simulink model "PMSM_PI_T"  (R2016a)
settings: Solver=ode23tb  StartTime=0.0  StopTime=1.4  FixedStep=Ts  MaxStep=0.0001  RelTol=1e-4
InitFcn:
  | Ts = 10e-6;
  | 
  | R = 0.958;
  | Ld = 5.25e-3;
  | Lq = 12e-3;
  | Pn = 4;
  | flux = 0.1827;
undefined symbols (not defined in the file): DiscIntNeverNeededParam
libraries: powerlib x13, simulink x2, powerlib_extras x2
settings Model: Creator=SUN  LastModifiedBy=Administrator
settings SolverCC: ZeroCrossControl=DisableAll
settings DataIOCC: LimitDataPoints=on  SaveFormat=Array  SignalLoggingSaveFormat=ModelDataLogs
settings OptimizationCC: ExpressionDepthLimit=2147483647  InitFltsAndDblsToZero=on
settings DebuggingCC: UnderspecifiedInitializationDetection=Classic  MergeDetectMultiDrivingBlocksExec=none  SolverPrmCheckMsg=warning  FcnCallInpInsideContextMsg=UseLocalSettings  StateNameClashWarn=warning
settings HardwareCC: ProdBitPerPointer=32  ProdLargestAtomicFloat=None  ProdIntDivRoundTo=Undefined  ProdEndianess=Unspecified  ProdWordSize=32  ProdHWDeviceType=32-bit Generic
settings ModelReferenceCC: PropagateSignalLabelsOutOfModel=off
settings GRTTargetCC: CombineOutputUpdateFcns=off  GRTInterface=on
settings ConfigComp: CovModelRefEnable=Off  CovSFcnEnable=off

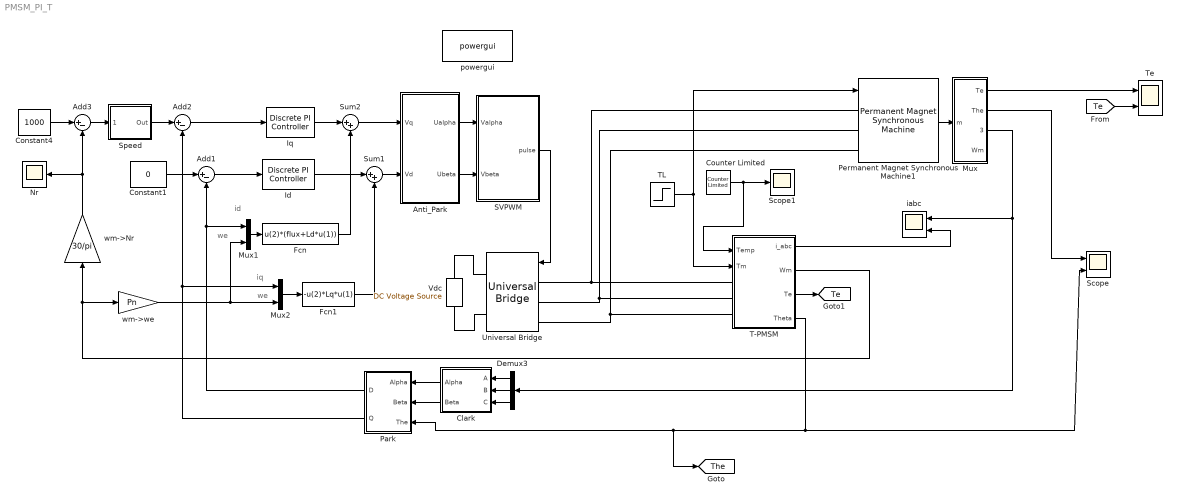
== system PMSM_PI_T ==
  note: iq
  note: we
  note: we
  note: id
  Add1 : Sum  Inputs=|+-
  Add2 : Sum  Inputs=|+-
  Add3 : Sum  Inputs=|+-
  Anti_Park : Subsystem
  Clark : Subsystem
  Constant1 : Constant  Value=0
  Constant4 : Constant  Value=1000
  Counter Limited : simulink/Sources/Counter Limited  uplimit=150  tsamp=0.0093
  Demux3 : Demux  Outputs=3
  Fcn : Fcn  Expr=u(2)*(flux+Ld*u(1))
  Fcn1 : Fcn  Expr=-u(2)*Lq*u(1)
  Id : powerlib_extras/Discrete  Control Blocks/Discrete PI Controller  Kp=Ld*1100  Ki=R*1100  Par_Limits=[311*0.9*sqrt(1/3) -311*0.9*sqrt(1/3)]  Init=0  Ts=Ts
  Iq : powerlib_extras/Discrete  Control Blocks/Discrete PI Controller  Kp=Lq*1100  Ki=R*1100  Par_Limits=[311*0.9*sqrt(1/3) -311*0.9*sqrt(1/3)]  Init=0  Ts=Ts
  Mux : Subsystem
  Mux1 : Mux  Inputs=2
  Mux2 : Mux  Inputs=2
  Nr : Scope
  Park : Subsystem
  Permanent Magnet Synchronous Machine1 : powerlib/Machines/Permanent Magnet Synchronous Machine  NbPhases=3  FluxDistribution=Sinusoidal  RotorType=Salient-pole  MechanicalLoad=Torque Tm  PresetModel=No  ShowDetailedParameters=on  MeasurementBus=off  Resistance=0.958  Inductance=8.5e-3  dqInductances=[5.25e-3,12e-3]  La=0.000835  MachineConstant=Flux linkage established by magnets (V.s)  Flux=0.1827  VoltageCst=132.5525  TorqueCst=1.0962  Flat=120  Mechanical=[0.003 0.008 4]  PolePairs=3  InitialConditions=[0,0, 0,0]  InitialConditions5ph=[0 0 0 0 0 0]  TsPowergui=0  TsBlock=-1  RefAngle=Aligned with phase A axis (original Park)
  SVPWM : Subsystem
  Scope : Scope  NumInputPorts=2
  Scope1 : Scope
  Speed : Subsystem  AncestorBlock=|  DialogController=POWERSYS.PowerSysDialog  mask(Discrete PI Controller){Kpw=0.14, Kiw=0.14*50, Ba=0.013, Par_Limits=[30 -30], Init=0, Ts=Ts}
      | powerlib_extras/Discrete 
      | Control Blocks/Discrete
      | PI Controller
      mask prompts: Kpw "Proportional gain (Kp):"; Kiw "Integral gain (Ki):"; Ba "feedback gain (Ba)"; Par_Limits "Output limits: [ Upper   Lower ]"; Init "Output initial value:"; Ts "Sample time:"
      mask help: This block implements a discrete PI controller.
      mask init:
      | UpperLimit=Par_Limits(1);
      | LowerLimit=Par_Limits(2);
      | power_initmask();
      mask Help: This block is part of a subset of blocks in the Extras library that does not have documentation associated with it, other than the block mask description.
      mask Display: disp('PI');
  Sum1 : Sum  Inputs=|++
  Sum2 : Sum  Inputs=|++
  T-PMSM : Subsystem
  TL : Step  Time=0.2  After=10  SampleTime=0
  Te : Scope  NumInputPorts=2
  Universal Bridge : powerlib/Power Electronics/Universal Bridge  Arms=3  SnubberResistance=1e5  SnubberCapacitance=inf  Device=IGBT / Diodes  Ron=1e-3  Lon=0  ForwardVoltages="[  0  0  ]"  ForwardVoltage=0  GTOparameters=[ 10e-6 , 20e-6 ]  IGBTparameters=[ 1e-6 , 2e-6 ]  Measurements=None  Measurements_2=None  converterType=Rectifier
  Vdc : powerlib/Electrical Sources/DC Voltage Source  Amplitude=311  Measurements=None
  iabc : Scope  NumInputPorts=2
  powergui : powerlib/powergui  SimulationMode=Continuous  SolverType=Tustin/Backward Euler (TBE)  SampleTime=Ts  frequency=60  SPID=off  DisableSnubberDevices=off  DisableRonSwitches=off  DisableVfSwitches=off  SwTol=0  DisplayEquations=off  Interpol=off  ExternalGateDelay=off  methode=off  Ts=0  FunctionMessages=off  echomessages=off  HookPort=off  EnableUseOfTLC=off  x0status=blocks  frequencyindice=0  Pbase=100e6  ErrMax=1e-4  Iterations=50  UnitsV=kV  UnitsW=MW  buscounter=0  RestoreLinks=warning  ResistiveCurrentMeasurement=off  Frange=[0:2:500]  Ylog=off  Xlog=on  ShowGrid=off  save=off  variable=ZData  structure=0  ZoomFFT=on  StartTime=0.0  cycles=1  DisplayStyle=1  fundamental=60  FreqAxis=off  MaxFrequency=1000  frequencyindicesteady=1  RmsSteady=1  display=off
  wm->Nr : Gain  Gain=30/pi
  wm->we : Gain  Gain=Pn
  tag scope: Te=global, The=global
  wires:
  TL/1 -> Permanent Magnet Synchronous Machine1/1, T-PMSM/2(Tm)
  Permanent Magnet Synchronous Machine1/1 -> Mux/1(m)
  Add3/1 -> Speed/1(Error)
  Constant4/1 -> Add3/1
  Fcn/1 -> Sum2/2
  Fcn1/1 -> Sum1/2
  Constant1/1 -> Add1/1
  Add1/1 -> Id/1
  wm->Nr/1 -> Add3/2, Nr/1
  Id/1 -> Sum1/1
  wm->we/1 -> Mux2/2, Mux1/2
  Mux1/1 -> Fcn/1
  Mux2/1 -> Fcn1/1
  Speed/1(Out) -> Add2/1
  Add2/1 -> Iq/1
  Iq/1 -> Sum2/1
  Sum2/1 -> Anti_Park/1(Vq)
  Sum1/1 -> Anti_Park/2(Vd)
  Mux/2(The) -> Scope/1
  SVPWM/1(pulse) -> Universal Bridge/1
  Mux/3(Iabc) -> Demux3/1, iabc/1
  Anti_Park/1(Ualpha) -> SVPWM/1(Valpha)
  Anti_Park/2(Ubeta) -> SVPWM/2(Vbeta)
  Clark/1(Alpha) -> Park/1(Alpha)
  Demux3/1 -> Clark/1(A)
  Demux3/2 -> Clark/2(B)
  Demux3/3 -> Clark/3(C)
  Clark/2(Beta) -> Park/2(Beta)
  Park/1(D) -> Mux1/1, Add1/2
  Park/2(Q) -> Mux2/1, Add2/2
  T-PMSM/1(i_abc) -> iabc/2
  T-PMSM/2(Wm) -> wm->we/1, wm->Nr/1
  T-PMSM/4(Theta) -> [The], Park/3(The), Scope/2
  T-PMSM/3(Te) -> [Te]
  [Te] -> Te/2
  Counter Limited/1 -> T-PMSM/1(Temp), Scope1/1
  Mux/1(Te) -> Te/1
  connections:
  Universal Bridge/RConn1 -- Vdc/RConn1
  Universal Bridge/RConn2 -- Vdc/LConn1
  Permanent Magnet Synchronous Machine1/LConn1 -- T-PMSM/LConn1 -- Universal Bridge/LConn1
  Permanent Magnet Synchronous Machine1/LConn2 -- Universal Bridge/LConn2 -- T-PMSM/LConn2
  Permanent Magnet Synchronous Machine1/LConn3 -- Universal Bridge/LConn3 -- T-PMSM/LConn3

== system PMSM_PI_T/Anti_Park ==
  Vq : Inport
  Vd : Inport  Port=2
  Fcn : Fcn  Expr=cos(u[1])*u[2]-sin(u[1])*u[3]
  Fcn1 : Fcn  Expr=sin(u[1])*u[2]+cos(u[1])*u[3]
  Mux1 : Mux  Inputs=3
  Ualpha : Outport
  Ubeta : Outport  Port=2
  wires:
  Fcn1/1 -> Ubeta/1
  Fcn/1 -> Ualpha/1
  Mux1/1 -> Fcn/1, Fcn1/1
  Vd/1 -> Mux1/2
  Vq/1 -> Mux1/3
  [The] -> Mux1/1

== system PMSM_PI_T/Clark ==
  A : Inport
  B : Inport  Port=2
  C : Inport  Port=3
  Mux : Mux  Inputs=3
  alpha : Fcn  Expr=(u(1)-0.5*(u(2)+u(3)))*2/3
  beta : Fcn  Expr=sqrt(3)/2*(u(2)-u(3))*2/3
  Alpha : Outport
  Beta : Outport  Port=2
  wires:
  alpha/1 -> Alpha/1
  B/1 -> Mux/2
  C/1 -> Mux/3
  A/1 -> Mux/1
  Mux/1 -> beta/1, alpha/1
  beta/1 -> Beta/1

== system PMSM_PI_T/Mux ==
  m : Inport
  Bus Selector : BusSelector  OutputSignals=Stator current is_a (A),Stator current is_b (A),Stator current is_c (A)
  Bus Selector1 : BusSelector  OutputSignals=Rotor speed wm (rad/s),Rotor angle thetam (rad),Electromagnetic torque Te (N*m)
  Mux : Mux  Inputs=3
  Te : Outport
  The : Outport  Port=2
  Iabc : Outport  Port=3
  Wm : Outport  Port=4
  wires:
  Bus Selector1/1 -> Wm/1  "<Rotor speed wm (rad/s)>"
  Bus Selector1/2 -> The/1  "<Rotor angle thetam (rad)>"
  Bus Selector1/3 -> Te/1  "<Electromagnetic torque Te (N*m)>"
  m/1 -> Bus Selector/1, Bus Selector1/1
  Bus Selector/2 -> Mux/2  "<Stator current is_b (A)>"
  Bus Selector/3 -> Mux/3  "<Stator current is_c (A)>"
  Bus Selector/1 -> Mux/1  "<Stator current is_a (A)>"
  Mux/1 -> Iabc/1

== system PMSM_PI_T/Park ==
  Alpha : Inport
  Beta : Inport  Port=2
  The : Inport  Port=3
  Mux : Mux  Inputs=3
  d : Fcn  Expr=u(1)*cos(u(3))+u(2)*sin(u(3))
  q : Fcn  Expr=-u(1)*sin(u(3))+u(2)*cos(u(3))
  D : Outport
  Q : Outport  Port=2
  wires:
  d/1 -> D/1
  Beta/1 -> Mux/2
  Alpha/1 -> Mux/1
  Mux/1 -> q/1, d/1
  q/1 -> Q/1
  The/1 -> Mux/3

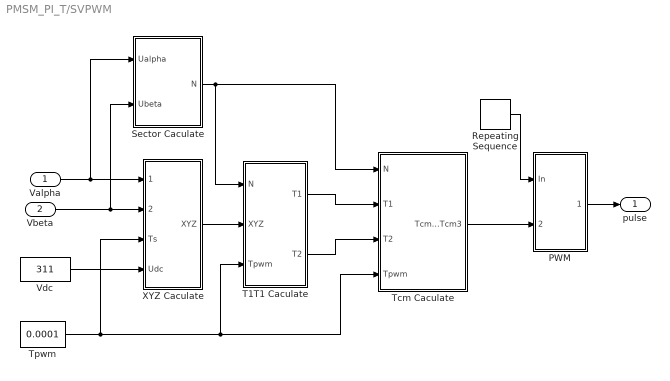
== system PMSM_PI_T/SVPWM ==
  Valpha : Inport
  Vbeta : Inport  Port=2
  PWM : Subsystem
  Repeating Sequence : simulink/Sources/Repeating Sequence  rep_seq_t=[0 0.00005 0.0001]  rep_seq_y=[0 0.00005 0]
  Sector Caculate : Subsystem
  T1T1 Caculate : Subsystem
  Tcm Caculate : Subsystem
  Tpwm : Constant  Value=0.0001
  Vdc : Constant  Value=311
  XYZ Caculate : Subsystem
  pulse : Outport
  wires:
  PWM/1(PWM) -> pulse/1
  Repeating Sequence/1 -> PWM/1(In)
  Vbeta/1 -> XYZ Caculate/2(Ubeta), Sector Caculate/2(Ubeta)
  T1T1 Caculate/1(T1) -> Tcm Caculate/2(T1)
  Valpha/1 -> XYZ Caculate/1(Ualpha), Sector Caculate/1(Ualpha)
  T1T1 Caculate/2(T2) -> Tcm Caculate/3(T2)
  Sector Caculate/1("N ") -> Tcm Caculate/1(N), T1T1 Caculate/1(N)
  XYZ Caculate/1(XYZ) -> T1T1 Caculate/2(XYZ)
  Tpwm/1 -> XYZ Caculate/3(Ts), Tcm Caculate/4(Tpwm), T1T1 Caculate/3(Tpwm)
  Vdc/1 -> XYZ Caculate/4(Udc)
  Tcm Caculate/1(Tcm1 Tcm2 Tcm3) -> PWM/2(Tcm123)

== system PMSM_PI_T/Speed ==
  note: Discrete PID Controller
  note: Pierre Giroux, Gilbert Sybille
      | Power System Simulation Laboratory
      | IREQ, Hydro-Quebc
  Error : Inport  SampleTime=Ts
  Discrete-Time Integrator : DiscreteIntegrator  InitialCondition=Init  SampleTime=Ts  LimitOutput=on  UpperSaturationLimit=UpperLimit  LowerSaturationLimit=LowerLimit  ICPrevOutput=DiscIntNeverNeededParam  ICPrevScaledInput=DiscIntNeverNeededParam
  Kp1 : Gain  Gain=Ba  SampleTime=Ts  SaturateOnIntegerOverflow=on  OutDataTypeStr=Inherit: Same as input  ParamDataTypeStr=Inherit: Same as input
  Kp4 : Gain  Gain=Kpw  SampleTime=Ts  SaturateOnIntegerOverflow=on  OutDataTypeStr=Inherit: Same as input  ParamDataTypeStr=Inherit: Same as input
  Kp5 : Gain  Gain=Kiw  SampleTime=Ts  SaturateOnIntegerOverflow=on  OutDataTypeStr=Inherit: Same as input  ParamDataTypeStr=Inherit: Same as input
  Saturation2 : Saturate  UpperLimit=UpperLimit  LowerLimit=LowerLimit  SampleTime=Ts
  Sum6 : Sum  Inputs=++-  SampleTime=Ts  SaturateOnIntegerOverflow=on  InputSameDT=on  OutDataTypeStr=Inherit: Same as first input
  Zero-Order Hold : ZeroOrderHold  SampleTime=Ts
  Out : Outport  SampleTime=Ts  InitialOutput=0
  wires:
  Error/1 -> Kp1/1, Kp5/1, Kp4/1
  Zero-Order Hold/1 -> Sum6/1
  Saturation2/1 -> Out/1
  Discrete-Time Integrator/1 -> Sum6/2
  Kp4/1 -> Zero-Order Hold/1
  Kp5/1 -> Discrete-Time Integrator/1
  Sum6/1 -> Saturation2/1
  Kp1/1 -> Sum6/3

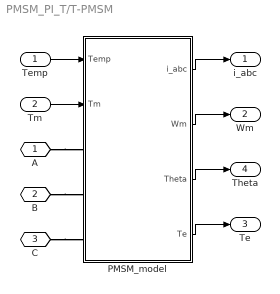
== system PMSM_PI_T/T-PMSM ==
  Temp : Inport
  Tm : Inport  Port=2
  PMSM_model : Subsystem  mask{Ld=5.25e-3, Lq=12e-3, Pn=4, flux=0.1827, B=0.008, J=0.003}
      mask prompts: Ld "d-Inductances(Ld)"; Lq "q-Inductances(Lq)"; Pn "pole pairs(Pn)"; flux "Flux linkage(flux)"; B "viscous damping(B)"; J "Inertia(J)"
      mask help: PMSM with the temperature
  A : PMIOPort  Port=1  Side=Left
  B : PMIOPort  Port=2  Side=Left
  C : PMIOPort  Port=3  Side=Left
  i_abc : Outport
  Wm : Outport  Port=2
  Te : Outport  Port=3
  Theta : Outport  Port=4
  wires:
  PMSM_model/1(i_abc) -> i_abc/1
  PMSM_model/2(Wm) -> Wm/1
  PMSM_model/4(Te) -> Te/1
  PMSM_model/3(Theta) -> Theta/1
  Tm/1 -> PMSM_model/2(Tm)
  Temp/1 -> PMSM_model/1(Temp)
  connections:
  B/RConn1 -- PMSM_model/LConn2
  A/RConn1 -- PMSM_model/LConn1
  C/RConn1 -- PMSM_model/LConn3

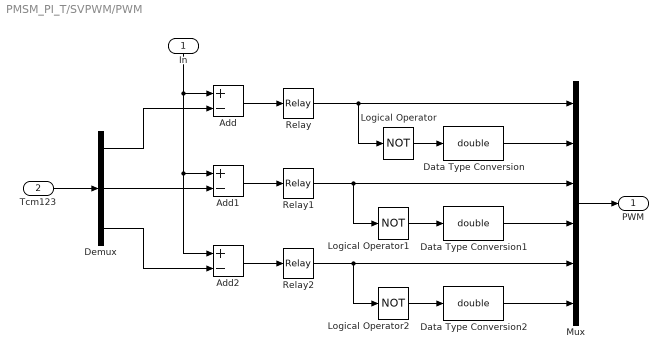
== system PMSM_PI_T/SVPWM/PWM ==
  In : Inport
  Tcm123 : Inport  Port=2
  Add : Sum  Inputs=+-
  Add1 : Sum  Inputs=+-
  Add2 : Sum  Inputs=+-
  Data Type Conversion : DataTypeConversion  OutDataTypeStr=double
  Data Type Conversion1 : DataTypeConversion  OutDataTypeStr=double
  Data Type Conversion2 : DataTypeConversion  OutDataTypeStr=double
  Demux : Demux  Outputs=3
  Logical Operator : Logic  Operator=NOT  AllPortsSameDT=off  OutDataTypeStr=boolean
  Logical Operator1 : Logic  Operator=NOT  AllPortsSameDT=off  OutDataTypeStr=boolean
  Logical Operator2 : Logic  Operator=NOT  AllPortsSameDT=off  OutDataTypeStr=boolean
  Mux : Mux  Inputs=6
  Relay : Relay  OffSwitchValue=-eps
  Relay1 : Relay  OffSwitchValue=-eps
  Relay2 : Relay  OffSwitchValue=-eps
  PWM : Outport
  wires:
  Demux/3 -> Add2/2
  Demux/2 -> Add1/2
  Demux/1 -> Add/2
  Relay2/1 -> Mux/5, Logical Operator2/1
  Relay1/1 -> Mux/3, Logical Operator1/1
  Relay/1 -> Logical Operator/1, Mux/1
  Mux/1 -> PWM/1
  Data Type Conversion/1 -> Mux/2
  Data Type Conversion1/1 -> Mux/4
  Data Type Conversion2/1 -> Mux/6
  Logical Operator2/1 -> Data Type Conversion2/1
  Logical Operator1/1 -> Data Type Conversion1/1
  Logical Operator/1 -> Data Type Conversion/1
  Add1/1 -> Relay1/1
  Add2/1 -> Relay2/1
  Add/1 -> Relay/1
  In/1 -> Add/1, Add2/1, Add1/1
  Tcm123/1 -> Demux/1

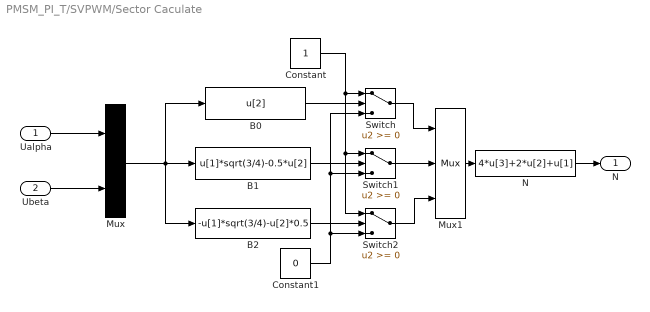
== system PMSM_PI_T/SVPWM/Sector Caculate ==
  Ualpha : Inport
  Ubeta : Inport  Port=2
  B0 : Fcn  Expr=u[2]
  B1 : Fcn  Expr=u[1]*sqrt(3/4)-0.5*u[2]
  B2 : Fcn  Expr=-u[1]*sqrt(3/4)-u[2]*0.5
  Constant : Constant
  Constant1 : Constant  Value=0
  Mux : Mux  Inputs=2
  Mux1 : Mux  Inputs=3
  N : Fcn  Expr=4*u[3]+2*u[2]+u[1]
  Switch : Switch
  Switch1 : Switch
  Switch2 : Switch
  "N " : Outport
  wires:
  Switch2/1 -> Mux1/3
  Switch/1 -> Mux1/1
  Ualpha/1 -> Mux/1
  Ubeta/1 -> Mux/2
  Mux/1 -> B2/1, B1/1, B0/1
  B0/1 -> Switch/2
  B1/1 -> Switch1/2
  B2/1 -> Switch2/2
  Constant/1 -> Switch/1, Switch2/1, Switch1/1
  Constant1/1 -> Switch/3, Switch1/3, Switch2/3
  Switch1/1 -> Mux1/2
  Mux1/1 -> N/1
  N/1 -> "N "/1

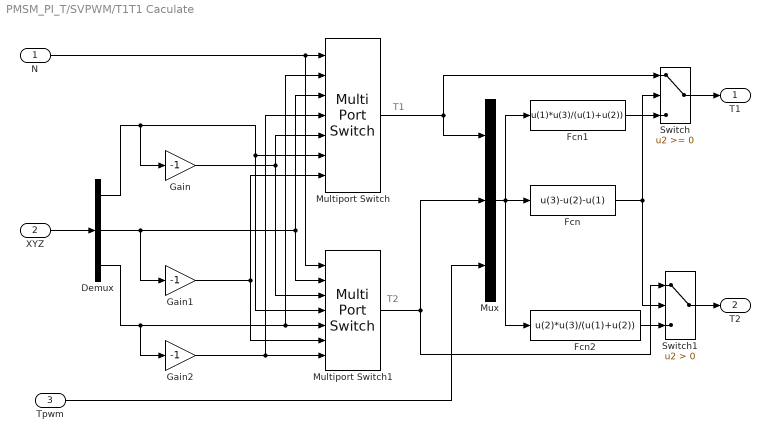
== system PMSM_PI_T/SVPWM/T1T1 Caculate ==
  note: T1
  note: T2
  N : Inport
  XYZ : Inport  Port=2
  Tpwm : Inport  Port=3
  Demux : Demux  Outputs=3
  Fcn : Fcn  Expr=u(3)-u(2)-u(1)
  Fcn1 : Fcn  Expr=u(1)*u(3)/(u(1)+u(2))
  Fcn2 : Fcn  Expr=u(2)*u(3)/(u(1)+u(2))
  Gain : Gain  Gain=-1
  Gain1 : Gain  Gain=-1
  Gain2 : Gain  Gain=-1
  Multiport Switch : MultiPortSwitch  Inputs=6
  Multiport Switch1 : MultiPortSwitch  Inputs=6
  Mux : Mux  Inputs=3
  Switch : Switch
  Switch1 : Switch  Criteria=u2 > Threshold
  T1 : Outport
  T2 : Outport  Port=2
  wires:
  Tpwm/1 -> Mux/3
  XYZ/1 -> Demux/1
  Switch1/1 -> T2/1
  Switch/1 -> T1/1
  Fcn2/1 -> Switch1/3
  Fcn1/1 -> Switch/3
  Fcn/1 -> Switch/2, Switch1/2
  Mux/1 -> Fcn1/1, Fcn/1, Fcn2/1
  Multiport Switch/1 -> Switch/1, Mux/1
  Multiport Switch1/1 -> Switch1/1, Mux/2
  N/1 -> Multiport Switch/1, Multiport Switch1/1
  Demux/2 -> Multiport Switch/3, Multiport Switch1/2, Gain1/1
  Demux/3 -> Multiport Switch1/5, Multiport Switch/2, Gain2/1
  Demux/1 -> Multiport Switch/6, Multiport Switch1/4, Gain/1
  Gain/1 -> Multiport Switch1/3, Multiport Switch/5
  Gain2/1 -> Multiport Switch/4, Multiport Switch1/7
  Gain1/1 -> Multiport Switch1/6, Multiport Switch/7

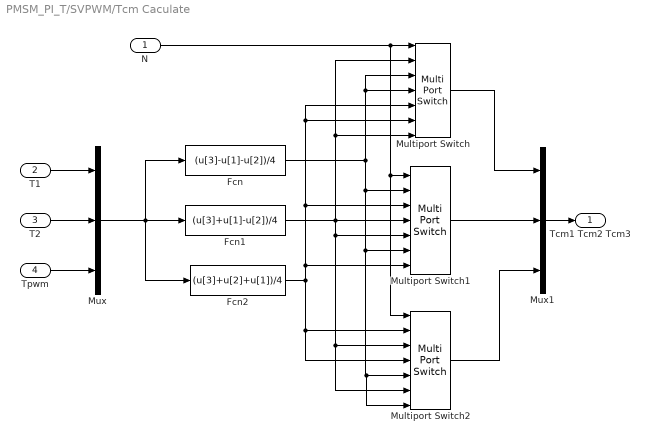
== system PMSM_PI_T/SVPWM/Tcm Caculate ==
  N : Inport
  T1 : Inport  Port=2
  T2 : Inport  Port=3
  Tpwm : Inport  Port=4
  Fcn : Fcn  Expr=(u[3]-u[1]-u[2])/4
  Fcn1 : Fcn  Expr=(u[3]+u[1]-u[2])/4
  Fcn2 : Fcn  Expr=(u[3]+u[2]+u[1])/4
  Multiport Switch : MultiPortSwitch  Inputs=6
  Multiport Switch1 : MultiPortSwitch  Inputs=6
  Multiport Switch2 : MultiPortSwitch  Inputs=6
  Mux : Mux  Inputs=3
  Mux1 : Mux  Inputs=3
  Tcm1 Tcm2 Tcm3 : Outport
  wires:
  Mux/1 -> Fcn2/1, Fcn/1, Fcn1/1
  Tpwm/1 -> Mux/3
  T2/1 -> Mux/2
  T1/1 -> Mux/1
  Multiport Switch2/1 -> Mux1/3
  Multiport Switch1/1 -> Mux1/2
  Multiport Switch/1 -> Mux1/1
  Mux1/1 -> Tcm1 Tcm2 Tcm3/1
  Fcn/1 -> Multiport Switch/3, Multiport Switch/4, Multiport Switch1/6, Multiport Switch2/5, Multiport Switch2/7, Multiport Switch1/2
  Fcn1/1 -> Multiport Switch1/5, Multiport Switch2/3, Multiport Switch2/6, Multiport Switch1/4, Multiport Switch/7, Multiport Switch/2
  Fcn2/1 -> Multiport Switch/5, Multiport Switch/6, Multiport Switch1/3, Multiport Switch1/7, Multiport Switch2/2, Multiport Switch2/4
  N/1 -> Multiport Switch2/1, Multiport Switch1/1, Multiport Switch/1

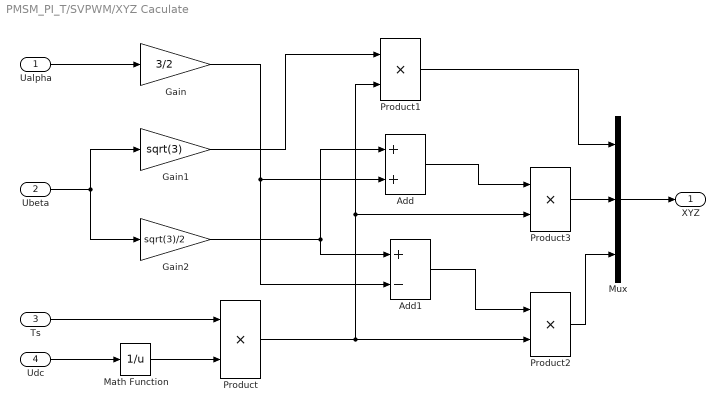
== system PMSM_PI_T/SVPWM/XYZ Caculate ==
  Ualpha : Inport
  Ubeta : Inport  Port=2
  Ts : Inport  Port=3
  Udc : Inport  Port=4
  Add : Sum
  Add1 : Sum  Inputs=+-
  Gain : Gain  Gain=3/2
  Gain1 : Gain  Gain=sqrt(3)
  Gain2 : Gain  Gain=sqrt(3)/2
  Math Function : Math  Operator=reciprocal  SaturateOnIntegerOverflow=on
  Mux : Mux  Inputs=3
  Product{,1..3} (4 alike) : Product  RndMeth=Zero
  XYZ : Outport
  wires:
  Mux/1 -> XYZ/1
  Product1/1 -> Mux/1
  Product3/1 -> Mux/2
  Product2/1 -> Mux/3
  Ualpha/1 -> Gain/1
  Ubeta/1 -> Gain2/1, Gain1/1
  Udc/1 -> Math Function/1
  Math Function/1 -> Product/2
  Ts/1 -> Product/1
  Gain1/1 -> Product1/1
  Product/1 -> Product2/2, Product1/2, Product3/2
  Gain/1 -> Add1/2, Add/2
  Gain2/1 -> Add/1, Add1/1
  Add1/1 -> Product2/1
  Add/1 -> Product3/1

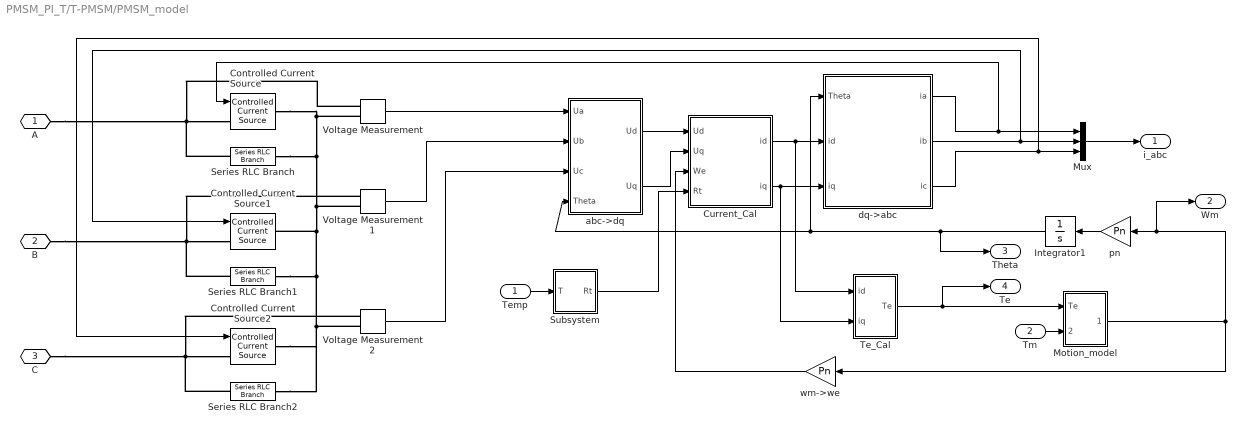
== system PMSM_PI_T/T-PMSM/PMSM_model ==
  Temp : Inport
  Tm : Inport  Port=2
  Controlled Current Source : powerlib/Electrical Sources/Controlled Current Source  Initialize=off  Source_Type=AC  Amplitude=0  Phase=0  Frequency=0  Measurements=None
  Controlled Current Source1 : powerlib/Electrical Sources/Controlled Current Source  Initialize=off  Source_Type=DC  Amplitude=0  Phase=0  Frequency=0  Measurements=None
  Controlled Current Source2 : powerlib/Electrical Sources/Controlled Current Source  Initialize=off  Source_Type=AC  Amplitude=0  Phase=0  Frequency=0  Measurements=None
  Current_Cal : Subsystem
  Integrator1 : Integrator
  Motion_model : Subsystem
  Mux : Mux  Inputs=3
  Series RLC Branch : powerlib/Elements/Series RLC Branch  LConnTagsString=__new0  RConnTagsString=__new0  BranchType=R  Resistance=100  Inductance=1e-3  SetiL0=off  InitialCurrent=0  Capacitance=1e-6  Setx0=off  InitialVoltage=0  Measurements=Branch voltage
  Series RLC Branch1 : powerlib/Elements/Series RLC Branch  LConnTagsString=__new0  RConnTagsString=__new0  BranchType=R  Resistance=1  Inductance=1e-3  SetiL0=off  InitialCurrent=0  Capacitance=1e-6  Setx0=off  InitialVoltage=0  Measurements=Branch voltage
  Series RLC Branch2 : powerlib/Elements/Series RLC Branch  LConnTagsString=__new0  RConnTagsString=__new0  BranchType=R  Resistance=1  Inductance=1e-3  SetiL0=off  InitialCurrent=0  Capacitance=1e-6  Setx0=off  InitialVoltage=0  Measurements=Branch voltage
  Subsystem : Subsystem
  Te_Cal : Subsystem
  Voltage Measurement : powerlib/Measurements/Voltage Measurement  PhasorSimulation=off  OutputType=Complex  PSBequivalent=0
  Voltage Measurement1 : powerlib/Measurements/Voltage Measurement  PhasorSimulation=off  OutputType=Complex  PSBequivalent=0
  Voltage Measurement2 : powerlib/Measurements/Voltage Measurement  PhasorSimulation=off  OutputType=Complex  PSBequivalent=0
  abc->dq : Subsystem
  dq->abc : Subsystem
  pn : Gain  Gain=Pn  SaturateOnIntegerOverflow=on  OutDataTypeStr=Inherit: Same as input  ParamDataTypeStr=Inherit: Same as input
  wm->we : Gain  Gain=Pn  SaturateOnIntegerOverflow=on  OutDataTypeStr=Inherit: Same as input  ParamDataTypeStr=Inherit: Same as input
  A : PMIOPort  Port=1  Side=Left
  B : PMIOPort  Port=2  Side=Left
  C : PMIOPort  Port=3  Side=Left
  i_abc : Outport
  Wm : Outport  Port=2
  Theta : Outport  Port=3
  Te : Outport  Port=4
  wires:
  Voltage Measurement/1 -> abc->dq/1(Ua)
  abc->dq/1(Ud) -> Current_Cal/1(Ud)
  abc->dq/2(Uq) -> Current_Cal/2(Uq)
  Current_Cal/1(id) -> Te_Cal/1(id), dq->abc/2(id)
  Current_Cal/2(iq) -> Te_Cal/2(iq), dq->abc/3(iq)
  Integrator1/1 -> abc->dq/4(Theta), dq->abc/1(Theta), Theta/1
  pn/1 -> Integrator1/1
  Voltage Measurement2/1 -> abc->dq/3(Uc)
  Voltage Measurement1/1 -> abc->dq/2(Ub)
  dq->abc/3(ic) -> Controlled Current Source2/1, Mux/3
  Mux/1 -> i_abc/1
  wm->we/1 -> Current_Cal/3(We)
  Motion_model/1(wm) -> wm->we/1, Wm/1, pn/1
  Te_Cal/1(Te) -> Te/1, Motion_model/1(Te)
  Tm/1 -> Motion_model/2(Tm)
  dq->abc/1(ia) -> Controlled Current Source/1, Mux/1
  dq->abc/2(ib) -> Controlled Current Source1/1, Mux/2
  Subsystem/1(Rt) -> Current_Cal/4(Rt)
  Temp/1 -> Subsystem/1(T)
  connections:
  A/RConn1 -- Voltage Measurement/LConn1 -- Series RLC Branch/LConn1 -- Controlled Current Source/LConn1
  B/RConn1 -- Series RLC Branch1/LConn1 -- Voltage Measurement1/LConn1 -- Controlled Current Source1/LConn1
  C/RConn1 -- Series RLC Branch2/LConn1 -- Voltage Measurement2/LConn1 -- Controlled Current Source2/LConn1
  Controlled Current Source/RConn1 -- Voltage Measurement/LConn2 -- Series RLC Branch/RConn1 -- Voltage Measurement1/LConn2 -- Voltage Measurement2/LConn2 -- Series RLC Branch2/RConn1 -- Controlled Current Source2/RConn1 -- Series RLC Branch1/RConn1 -- Controlled Current Source1/RConn1

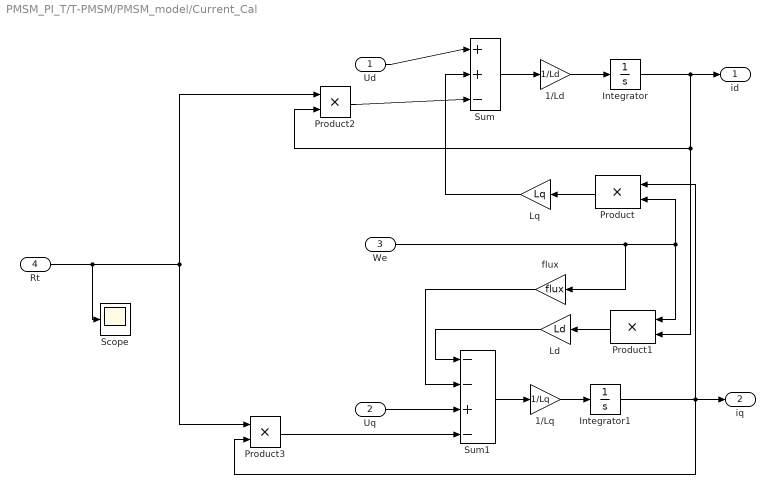
== system PMSM_PI_T/T-PMSM/PMSM_model/Current_Cal ==
  Ud : Inport
  Uq : Inport  Port=2
  We : Inport  Port=3
  Rt : Inport  Port=4
  1/Ld : Gain  Gain=1/Ld  SaturateOnIntegerOverflow=on  OutDataTypeStr=Inherit: Same as input  ParamDataTypeStr=Inherit: Same as input
  1/Lq : Gain  Gain=1/Lq  SaturateOnIntegerOverflow=on  OutDataTypeStr=Inherit: Same as input  ParamDataTypeStr=Inherit: Same as input
  Integrator : Integrator  InitialCondition=0.01
  Integrator1 : Integrator
  Ld : Gain  Gain=Ld  SaturateOnIntegerOverflow=on  OutDataTypeStr=Inherit: Same as input  ParamDataTypeStr=Inherit: Same as input
  Lq : Gain  Gain=Lq  SaturateOnIntegerOverflow=on  OutDataTypeStr=Inherit: Same as input  ParamDataTypeStr=Inherit: Same as input
  Product : Product  SaturateOnIntegerOverflow=on  OutDataTypeStr=Inherit: Same as first input
  Product1 : Product  SaturateOnIntegerOverflow=on  OutDataTypeStr=Inherit: Same as first input
  Product2 : Product
  Product3 : Product
  Scope : Scope
  Sum : Sum  Inputs=|++-  SaturateOnIntegerOverflow=on
  Sum1 : Sum  Inputs=--+-  SaturateOnIntegerOverflow=on
  flux : Gain  Gain=flux  SaturateOnIntegerOverflow=on  OutDataTypeStr=Inherit: Same as input  ParamDataTypeStr=Inherit: Same as input
  id : Outport
  iq : Outport  Port=2
  wires:
  Ud/1 -> Sum/1
  Sum/1 -> 1/Ld/1
  1/Ld/1 -> Integrator/1
  Integrator/1 -> Product1/2, Product2/2, id/1
  Product/1 -> Lq/1
  Lq/1 -> Sum/2
  We/1 -> Product/2, Product1/1, flux/1
  Product3/1 -> Sum1/4
  1/Lq/1 -> Integrator1/1
  Sum1/1 -> 1/Lq/1
  Integrator1/1 -> Product3/2, Product/1, iq/1
  Product1/1 -> Ld/1
  Ld/1 -> Sum1/1
  Uq/1 -> Sum1/3
  flux/1 -> Sum1/2
  Product2/1 -> Sum/3
  Rt/1 -> Scope/1, Product3/1, Product2/1

== system PMSM_PI_T/T-PMSM/PMSM_model/Motion_model ==
  Te : Inport
  Tm : Inport  Port=2
  1/J : Gain  Gain=1/J  SaturateOnIntegerOverflow=on  OutDataTypeStr=Inherit: Same as input  ParamDataTypeStr=Inherit: Same as input
  B : Gain  Gain=B  SaturateOnIntegerOverflow=on  OutDataTypeStr=Inherit: Same as input  ParamDataTypeStr=Inherit: Same as input
  Integrator : Integrator
  Sum1 : Sum  Inputs=|+--  SaturateOnIntegerOverflow=on
  wm : Outport
  wires:
  Tm/1 -> Sum1/3
  Sum1/1 -> 1/J/1
  B/1 -> Sum1/2
  1/J/1 -> Integrator/1
  Te/1 -> Sum1/1
  Integrator/1 -> B/1, wm/1

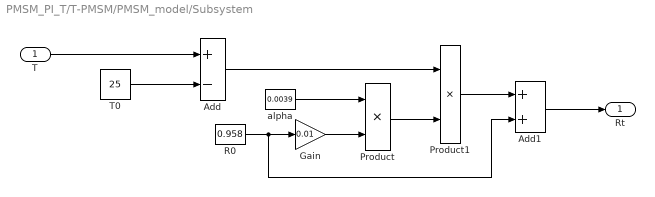
== system PMSM_PI_T/T-PMSM/PMSM_model/Subsystem ==
  T : Inport
  Add : Sum  Inputs=+-
  Add1 : Sum
  Gain : Gain  Gain=0.01
  Product : Product
  Product1 : Product
  R0 : Constant  Value=0.958
  T0 : Constant  Value=25
  alpha : Constant  Value=0.0039
  Rt : Outport
  wires:
  Gain/1 -> Product/2
  R0/1 -> Add1/2, Gain/1
  alpha/1 -> Product/1
  T/1 -> Add/1
  Add/1 -> Product1/1
  T0/1 -> Add/2
  Add1/1 -> Rt/1
  Product1/1 -> Add1/1
  Product/1 -> Product1/2

== system PMSM_PI_T/T-PMSM/PMSM_model/Te_Cal ==
  id : Inport
  iq : Inport  Port=2
  1.5*极对数 : Gain  Gain=1.5*Pn
  Ld-Lq : Gain  Gain=Ld-Lq  SaturateOnIntegerOverflow=on  OutDataTypeStr=Inherit: Same as input  ParamDataTypeStr=Inherit: Same as input
  Product : Product  SaturateOnIntegerOverflow=on  OutDataTypeStr=Inherit: Same as first input
  Sum : Sum  SaturateOnIntegerOverflow=on
  flux : Gain  Gain=flux  SaturateOnIntegerOverflow=on  OutDataTypeStr=Inherit: Same as input  ParamDataTypeStr=Inherit: Same as input
  Te : Outport
  wires:
  id/1 -> Product/1
  Ld-Lq/1 -> Sum/1
  Product/1 -> Ld-Lq/1
  flux/1 -> Sum/2
  iq/1 -> flux/1, Product/2
  Sum/1 -> 1.5*极对数/1
  1.5*极对数/1 -> Te/1

== system PMSM_PI_T/T-PMSM/PMSM_model/abc->dq ==
  Ua : Inport
  Ub : Inport  Port=2
  Uc : Inport  Port=3
  Theta : Inport  Port=4
  Mux : Mux
  d : Fcn  Expr=(u(1)*cos(u(4))+u(2)*cos(u(4)-2/3*pi)+u(3)*cos(u(4)+2/3*pi))*2/3
  q : Fcn  Expr=-(u(1)*sin(u(4))+u(2)*sin(u(4)-2/3*pi)+u(3)*sin(u(4)+2/3*pi))*2/3
  Ud : Outport
  Uq : Outport  Port=2
  wires:
  Mux/1 -> q/1, d/1
  Ub/1 -> Mux/2
  d/1 -> Ud/1
  Theta/1 -> Mux/4
  Uc/1 -> Mux/3
  q/1 -> Uq/1
  Ua/1 -> Mux/1

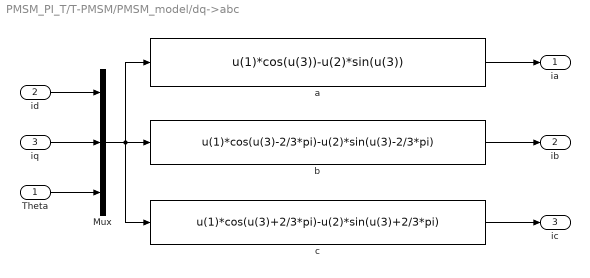
== system PMSM_PI_T/T-PMSM/PMSM_model/dq->abc ==
  Theta : Inport
  id : Inport  Port=2
  iq : Inport  Port=3
  Mux : Mux  Inputs=3
  a : Fcn  Expr=u(1)*cos(u(3))-u(2)*sin(u(3))
  b : Fcn  Expr=u(1)*cos(u(3)-2/3*pi)-u(2)*sin(u(3)-2/3*pi)
  c : Fcn  Expr=u(1)*cos(u(3)+2/3*pi)-u(2)*sin(u(3)+2/3*pi)
  ia : Outport
  ib : Outport  Port=2
  ic : Outport  Port=3
  wires:
  b/1 -> ib/1
  Theta/1 -> Mux/3
  a/1 -> ia/1
  id/1 -> Mux/1
  iq/1 -> Mux/2
  Mux/1 -> c/1, a/1, b/1
  c/1 -> ic/1
